simulink model "Offline_FLIP_FLOP"  (R2022b)
settings: Solver=VariableStepAuto  StartTime=0.0  StopTime=10.0  RelTol=1e-3
values from neighbouring files (symbols this model uses):
  alpha_max = 15    [Flip_Flop_StartUp.m]
  theta_max = 45    [Flip_Flop_StartUp.m]
libraries: simulink x3, dspsrcs4 x2, simulink_extras x1
settings Model: Creator=albif  LastModifiedBy=albif

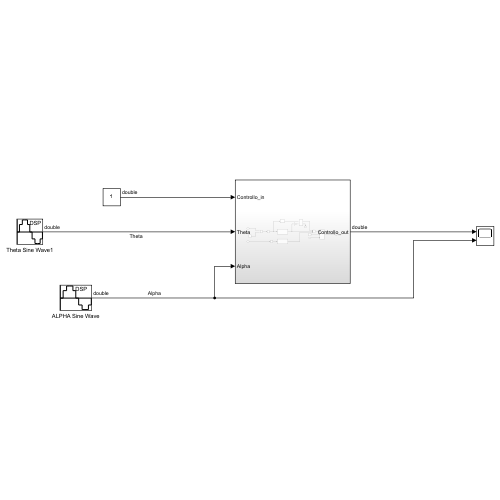
[thumbnail: Simulink's stored preview of the top-level diagram]
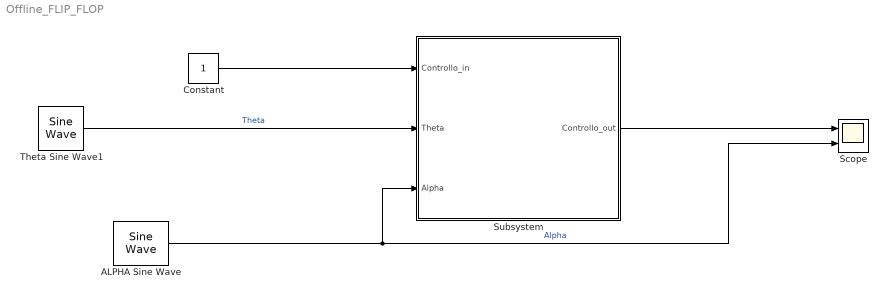
== system Offline_FLIP_FLOP ==
  ALPHA Sine Wave : dspsrcs4/Sine Wave  Amplitude=0.3  Frequency=0.3  Phase=pi/4  SampleMode=Discrete  OutComplex=Real  CompMethod=Trigonometric fcn  TableSize=Speed  SampleTime=1/1000  SamplesPerFrame=1  ResetState=Restart at time zero  OutputFrames=off  dataType=double  wordLen=16  udDataType=sfix(16)  fracBitsMode=Best precision  numFracBits=15  OutDataTypeStr=double  LastOutDataTypeStr=double
  Constant : Constant
  Scope : Scope  NumInputPorts=2
  Subsystem : Subsystem
  Theta Sine Wave1 : dspsrcs4/Sine Wave  Amplitude=0.8  Frequency=0.5  Phase=pi/4  SampleMode=Discrete  OutComplex=Real  CompMethod=Trigonometric fcn  TableSize=Speed  SampleTime=1/1000  SamplesPerFrame=1  ResetState=Restart at time zero  OutputFrames=off  dataType=double  wordLen=16  udDataType=sfix(16)  fracBitsMode=Best precision  numFracBits=15  OutDataTypeStr=double  LastOutDataTypeStr=double
  wires:
  ALPHA Sine Wave/1 -> Subsystem/3(Alpha), Scope/2  "Alpha"
  Constant/1 -> Subsystem/1(Controllo_in)
  Subsystem/1(Controllo_out) -> Scope/1
  Theta Sine Wave1/1 -> Subsystem/2(Theta)  "Theta"

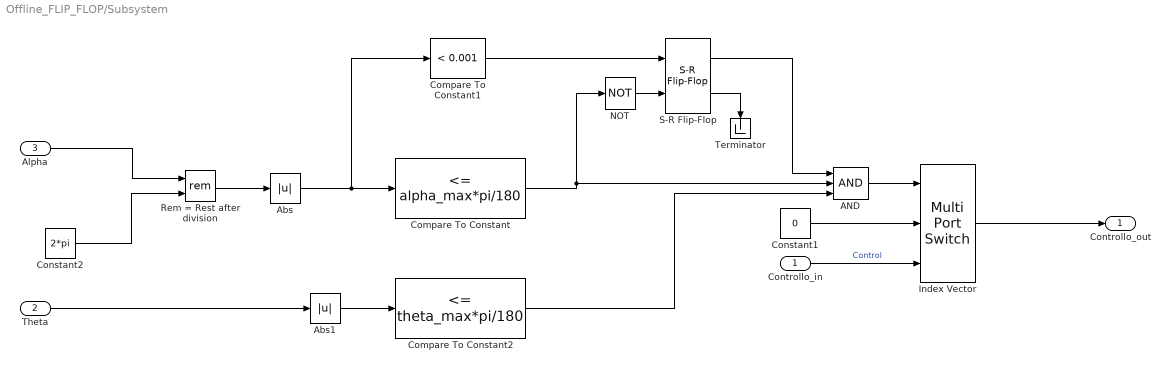
== system Offline_FLIP_FLOP/Subsystem ==
  Controllo_in : Inport
  Theta : Inport  Port=2
  Alpha : Inport  Port=3
  AND : Logic  Inputs=3  IconShape=distinctive  AllPortsSameDT=off  OutDataTypeStr=boolean
  Abs : Abs  SaturateOnIntegerOverflow=off
  Abs1 : Abs  SaturateOnIntegerOverflow=off
  Compare To Constant : simulink/Logic and Bit Operations/Compare To Constant  relop=<=  const=alpha_max*pi/180  OutDataTypeStr=boolean
  Compare To Constant1 : simulink/Logic and Bit Operations/Compare To Constant  relop=<  const=0.001  OutDataTypeStr=boolean
  Compare To Constant2 : simulink/Logic and Bit Operations/Compare To Constant  relop=<=  const=theta_max*pi/180  OutDataTypeStr=boolean
  Constant1 : Constant  Value=0
  Constant2 : Constant  Value=2*pi
  Index Vector : MultiPortSwitch  DataPortOrder=Zero-based contiguous  Inputs=2  zeroidx=on  SaturateOnIntegerOverflow=off  InputSameDT=off
  NOT : Logic  Operator=NOT  IconShape=distinctive  AllPortsSameDT=off  OutDataTypeStr=boolean
  Rem = Rest after division : Math  Operator=rem
  S-R Flip-Flop : simulink_extras/Flip Flops/S-R Flip-Flop  initial_condition=0
  Terminator : Terminator
  Controllo_out : Outport
  wires:
  NOT/1 -> S-R Flip-Flop/2
  Compare To Constant/1 -> AND/2, NOT/1
  Alpha/1 -> Rem = Rest after division/1
  Controllo_in/1 -> Index Vector/3  "Control"
  Constant1/1 -> Index Vector/2
  Rem = Rest after division/1 -> Abs/1
  S-R Flip-Flop/1 -> AND/1
  Constant2/1 -> Rem = Rest after division/2
  AND/1 -> Index Vector/1
  Abs/1 -> Compare To Constant/1, Compare To Constant1/1
  Compare To Constant1/1 -> S-R Flip-Flop/1
  Index Vector/1 -> Controllo_out/1
  S-R Flip-Flop/2 -> Terminator/1
  Theta/1 -> Abs1/1
  Abs1/1 -> Compare To Constant2/1
  Compare To Constant2/1 -> AND/3
